simulink model "working_motor"  (R2017a)
settings: Solver=FixedStepAuto  StartTime=0.0  StopTime=inf  RelTol=1e-3  EnableMultiTasking=on
libraries: simulink x4, hdlsllib x3
settings Model: Creator=hyang344  LastModifiedBy=hyang344
settings SolverCC: AutoInsertRateTranBlk=on
settings OptimizationCC: BlockReduction=off  ConditionallyExecuteInputs=off  DefaultParameterBehavior=Inlined
settings DebuggingCC: AlgebraicLoopMsg=error  SingleTaskRateTransMsg=error
settings HardwareCC: ProdBitPerPointer=32  ProdBitPerSizeT=32  ProdBitPerPtrDiffT=32  ProdLargestAtomicFloat=None  ProdIntDivRoundTo=Undefined  ProdEndianess=Unspecified  ProdWordSize=32  ProdHWDeviceType=ASIC/FPGA->ASIC/FPGA  ProdEqTarget=off

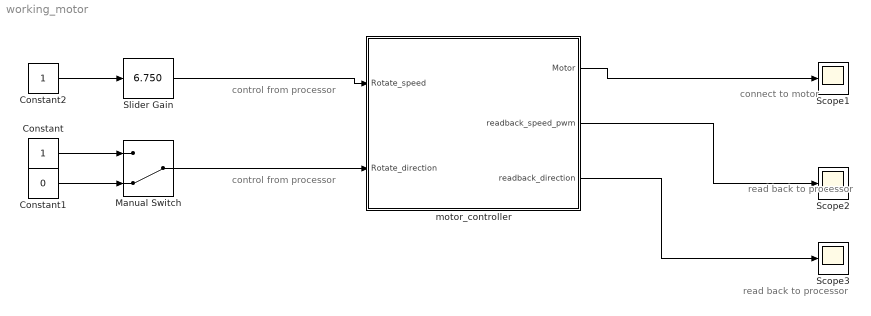
== system working_motor ==
  note: control from
      | processor
  note: read back to
      | processor
  note: control from
      | processor
  note: connect to
      | motor
  note: read back to
      | processor
  Constant : Constant  OutDataTypeStr=boolean
  Constant1 : Constant  Value=0  OutDataTypeStr=boolean
  Constant2 : Constant  OutDataTypeStr=fixdt(0, 4, 0)  SampleTime=0.1
  Manual Switch : ManualSwitch  CurrentSetting=0
  Scope1 : Scope
  Scope2 : Scope
  Scope3 : Scope
  Slider Gain : simulink/Math Operations/Slider Gain  gain=6.750  low=0  high=15
  motor_controller : Subsystem  TreatAsAtomicUnit=on
  wires:
  Constant1/1 -> Manual Switch/2
  Slider Gain/1 -> motor_controller/1(Rotate_speed)
  Constant2/1 -> Slider Gain/1
  motor_controller/1(Motor) -> Scope1/1
  Constant/1 -> Manual Switch/1
  Manual Switch/1 -> motor_controller/2(Rotate_direction)
  motor_controller/2(readback_speed_pwm) -> Scope2/1
  motor_controller/3("readback_direction ") -> Scope3/1

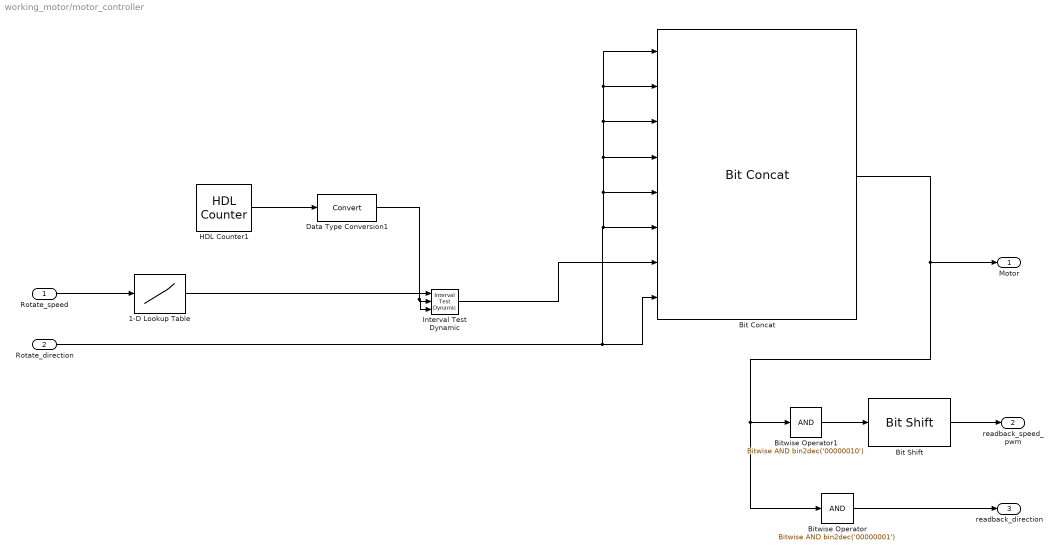
== system working_motor/motor_controller ==
  Rotate_speed : Inport  OutDataTypeStr=fixdt(0, 4, 0)
  Rotate_direction : Inport  Port=2  OutDataTypeStr=boolean
  1-D Lookup Table : Lookup_n-D  NumberOfTableDimensions=1  BreakpointsForDimension1=[0:15]  IndexSearchMethod=Evenly spaced points  Table=25000 * [0.25:0.05:1]  TableDataTypeStr=fixdt(0, 24, 0)  InterpMethod=Flat  DiagnosticForOutOfRangeInput=Error  OutDataTypeStr=fixdt(0, 24, 0)  RndMeth=Simplest  InputSameDT=on
  Bit Concat : hdlsllib/HDL Operations/Bit Concat  numInputs=8
      settings: SourceProductName=HDL Coder  SourceProductBaseCode=HD
  Bit Shift : hdlsllib/HDL Operations/Bit Shift  mode=Shift Right Logical  N=1
      settings: SourceProductName=HDL Coder  SourceProductBaseCode=HD
  Bitwise Operator : simulink/Logic and Bit Operations/Bitwise Operator  logicop=AND  UseBitMask=on  BitMask=bin2dec('00000001')  BitMaskRealWorld=Stored Integer
  Bitwise Operator1 : simulink/Logic and Bit Operations/Bitwise Operator  logicop=AND  UseBitMask=on  BitMask=bin2dec('00000010')  BitMaskRealWorld=Stored Integer
  Data Type Conversion1 : DataTypeConversion
  HDL Counter1 : hdlsllib/HDL Operations/HDL Counter  CountType=Count limited  CountInit=0  CountStep=1  CountMax=25000  CountFromType=Initial value  CountFrom=0  CountResetPort=off  CountLoadPort=off  CountEnbPort=off  CountDirPort=off  CountDataType=Unsigned  CountWordLen=16  CountFracLen=0  CountSampTime=0.1
      settings: SourceProductName=HDL Coder  SourceProductBaseCode=HD
  Interval Test Dynamic : simulink/Logic and Bit Operations/Interval Test Dynamic  IntervalClosedRight=on  IntervalClosedLeft=on  OutDataTypeStr=boolean
      settings: SourceProductName=Simulink  SourceProductBaseCode=SL
  Motor : Outport
  readback_speed_pwm : Outport  Port=2
  "readback_direction " : Outport  Port=3
  wires:
  Rotate_speed/1 -> 1-D Lookup Table/1
  1-D Lookup Table/1 -> Interval Test Dynamic/1
  Rotate_direction/1 -> Bit Concat/1, Bit Concat/2, Bit Concat/3, Bit Concat/4, Bit Concat/5, Bit Concat/6, Bit Concat/8
  HDL Counter1/1 -> Data Type Conversion1/1
  Data Type Conversion1/1 -> Interval Test Dynamic/3, Interval Test Dynamic/2
  Interval Test Dynamic/1 -> Bit Concat/7
  Bit Shift/1 -> readback_speed_pwm/1
  Bitwise Operator/1 -> "readback_direction "/1
  Bitwise Operator1/1 -> Bit Shift/1
  Bit Concat/1 -> Bitwise Operator1/1, Bitwise Operator/1, Motor/1
